simulink model "lqr_nl"  (R2024b)
settings: Solver=VariableStepAuto  StartTime=0.0  StopTime=params.simtime  RelTol=1e-3
values from neighbouring files (symbols this model uses):
  params = parameters()    [lqr_STM_compare.m]    (also in lqr_compare.m; lqr_main_isolated.m)
undefined symbols (not defined in the file or in its folder): nl_model
settings Model: Creator=ben83  LastModifiedBy=ben
settings RTWCC: GPUComputeCapability=3.5

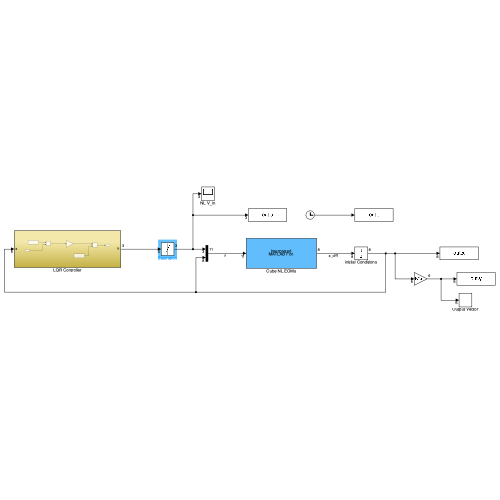
[thumbnail: Simulink's stored preview of the top-level diagram]
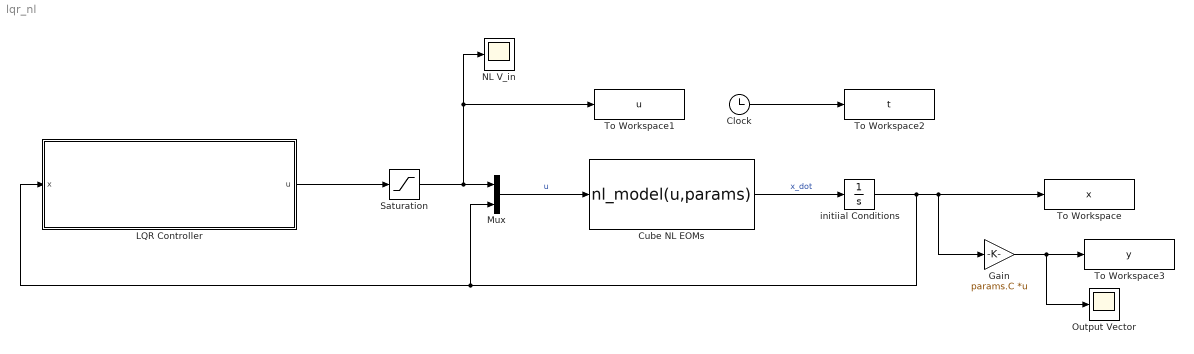
== system lqr_nl ==
  Clock : Clock
  Cube NL EOMs : MATLABFcn  MATLABFcn=nl_model(u,params)  OutputDimensions=8
  Gain : Gain  Gain=params.C  Multiplication=Matrix(K*u)
  LQR Controller : Subsystem
  Mux : Mux  Inputs=2
  NL V_in : Scope
  Output Vector : Scope
  Saturation : Saturate  UpperLimit=10.8  LowerLimit=-10.8
  To Workspace : ToWorkspace  VariableName=x  SampleTime=-1
  To Workspace1 : ToWorkspace  VariableName=u  SampleTime=-1
  To Workspace2 : ToWorkspace  VariableName=t  SampleTime=-1
  To Workspace3 : ToWorkspace  VariableName=y  SampleTime=-1
  initiial Conditions : Integrator  InitialCondition=params.ic
  wires:
  Cube NL EOMs/1 -> initiial Conditions/1  "x_dot"
  Mux/1 -> Cube NL EOMs/1  "u"
  Clock/1 -> To Workspace2/1
  initiial Conditions/1 -> LQR Controller/1(x), Mux/2, Gain/1, To Workspace/1
  Gain/1 -> Output Vector/1, To Workspace3/1
  Saturation/1 -> NL V_in/1, To Workspace1/1, Mux/1
  LQR Controller/1(u) -> Saturation/1

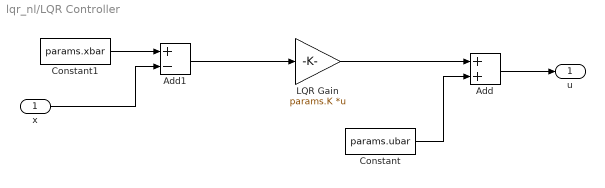
== system lqr_nl/LQR Controller ==
  x : Inport
  Add : Sum
  Add1 : Sum  Inputs=+-
  Constant : Constant  Value=params.ubar
  Constant1 : Constant  Value=params.xbar
  LQR Gain : Gain  Gain=params.K  Multiplication=Matrix(K*u)
  u : Outport
  wires:
  LQR Gain/1 -> Add/1
  Add/1 -> u/1
  x/1 -> Add1/2
  Constant1/1 -> Add1/1
  Constant/1 -> Add/2
  Add1/1 -> LQR Gain/1
